simulink model "pid_simulink_with_r_and_d"  (R2015a)
settings: Solver=ode45  SolverMode=SingleTasking  StartTime=0.0  StopTime=simu.time  RelTol=1e-3
values from neighbouring files (symbols this model uses):
  plant = tf([10],[tau 1])    [mpc_period_with_abitary_reference.m]
undefined symbols (not defined in the file or in its folder): plant_ref, simu
libraries: simulink x1
settings Model: CovSFcnEnable=off  ExtModeTrigMode=oneshot  ExtModeArmWhenConnect=off  Creator=The MathWorks Inc.  LastModifiedBy=Xiaotian
settings DataIOCC: LimitDataPoints=off  SaveOutput=off  SignalLogging=off  DSMLogging=off  SaveTime=off  SignalLoggingName=sigsOut
settings OptimizationCC: BooleanDataType=off  ExpressionDepthLimit=2147483647  InitFltsAndDblsToZero=on
settings DebuggingCC: SaveWithParameterizedLinksMsg=none  UnderspecifiedInitializationDetection=Classic  MergeDetectMultiDrivingBlocksExec=none  SignalResolutionControl=TryResolveAllWithWarning  MultiTaskDSMMsg=warning  MultiTaskCondExecSysMsg=none  IntegerOverflowMsg=none  FcnCallInpInsideContextMsg=UseLocalSettings  StateNameClashWarn=warning  IntegerSaturationMsg=none
settings HardwareCC: TargetUnknown=on
settings GRTTargetCC: TargetFcnLib=ansi_tfl_tmw.mat  CombineOutputUpdateFcns=off  GRTInterface=on

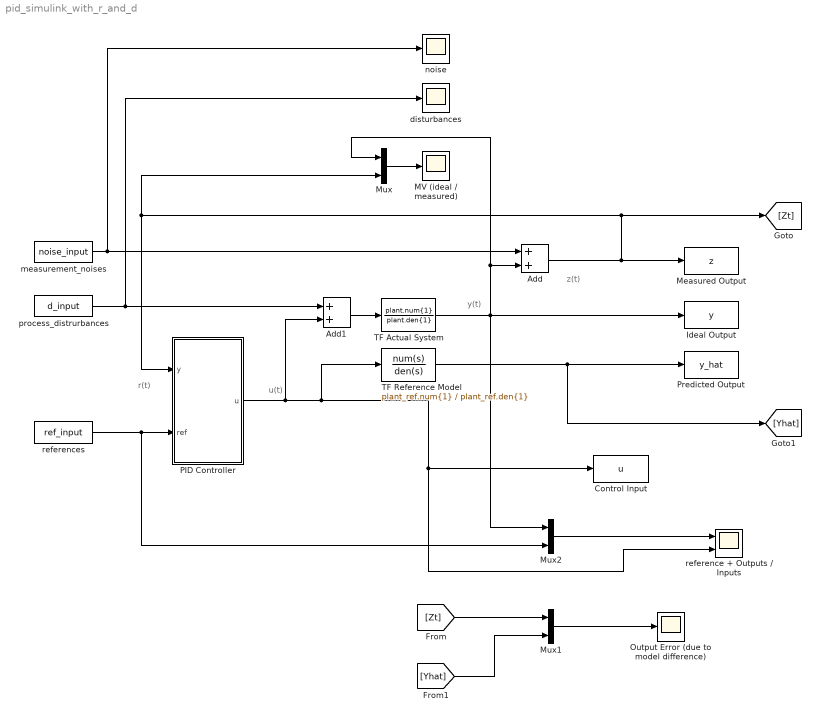
== system pid_simulink_with_r_and_d ==
  note: r(t)
  note: u(t)
  note: y(t)
  note: z(t)
  Add : Sum
  Add1 : Sum
  Control Input : ToWorkspace  VariableName=u  SampleTime=simu.samlping_time
      settings: MaxDataPoints=Inf
  Ideal Output : ToWorkspace  VariableName=y  SampleTime=simu.samlping_time
      settings: MaxDataPoints=Inf
  MV (ideal / measured) : Scope
      settings: TimeRange=10  YMin=-1.5  YMax=1.75  DataFormat=Structure
  Measured Output : ToWorkspace  VariableName=z  SampleTime=simu.samlping_time
      settings: MaxDataPoints=Inf
  Mux : Mux  Inputs=2
  Mux1 : Mux  Inputs=2
  Mux2 : Mux  Inputs=2
  Output Error (due to model difference) : Scope
      settings: TimeRange=10  YMin=-29.95  YMax=-29.6  SaveName=ScopeData2  DataFormat=Structure  SampleInput=on  SampleTime=simu.samlping_time
  PID Controller : Subsystem
  Predicted Output : ToWorkspace  VariableName=y_hat  SampleTime=simu.samlping_time
      settings: MaxDataPoints=Inf
  TF Actual System : TransferFcn  Numerator=plant.num{1}  Denominator=plant.den{1}
  TF Reference Model : TransferFcn  Numerator=plant_ref.num{1}  Denominator=plant_ref.den{1}
  disturbances : Scope
      settings: TimeRange=10  YMin=-29.95  YMax=-29.6  SaveName=ScopeData4  DataFormat=Structure  SampleInput=on  SampleTime=simu.samlping_time
  measurement_noises : FromWorkspace  VariableName=noise_input  SampleTime=0
  noise : Scope
      settings: TimeRange=10  YMin=-29.95  YMax=-29.6  SaveName=ScopeData3  DataFormat=Structure  SampleInput=on  SampleTime=simu.samlping_time
  process_distrurbances : FromWorkspace  VariableName=d_input  SampleTime=0
  reference + Outputs / Inputs : Scope  NumInputPorts=2
      settings: TimeRange=10  YMin=-2e+58~-6e+59  YMax=6.000000000000001e+58~2e+59  DataFormat=Structure  SampleInput=on  SampleTime=simu.samlping_time
  references : FromWorkspace  VariableName=ref_input  SampleTime=0
  wires:
  PID Controller/1(u) -> Add1/2, Control Input/1, reference + Outputs / Inputs/2, TF Reference Model/1
  TF Actual System/1 -> Mux2/1, Mux/1, Add/2, Ideal Output/1
  references/1 -> Mux2/2, PID Controller/2(ref)
  Add/1 -> Measured Output/1, PID Controller/1(y), Mux/2, [Zt]
  measurement_noises/1 -> noise/1, Add/1
  Add1/1 -> TF Actual System/1
  process_distrurbances/1 -> disturbances/1, Add1/1
  Mux/1 -> MV (ideal / measured)/1
  TF Reference Model/1 -> [Yhat], Predicted Output/1
  Mux1/1 -> Output Error (due to model difference)/1
  [Zt] -> Mux1/1
  [Yhat] -> Mux1/2
  Mux2/1 -> reference + Outputs / Inputs/1

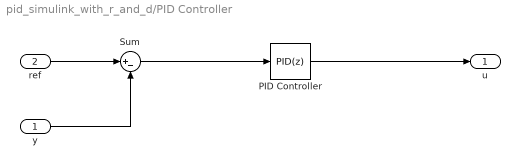
== system pid_simulink_with_r_and_d/PID Controller ==
  y : Inport
  ref : Inport  Port=2
  PID Controller : simulink/Continuous/PID Controller  Controller=PID  TimeDomain=Discrete-time  SampleTime=0.035  IntegratorMethod=Forward Euler  FilterMethod=Forward Euler  Form=Parallel  UseFilter=on  ControllerParametersSource=internal  P=10  I=1  D=0  N=10  InitialConditionSource=internal  InitialConditionForIntegrator=0  InitialConditionForFilter=0  ExternalReset=none  LimitOutput=off  UpperSaturationLimit=inf  LowerSaturationLimit=-inf  LinearizeAsGain=on  AntiWindupMode=none  Kb=1  TrackingMode=off  Kt=1  PParamMin=[]  PParamMax=[]  IParamMin=[]  IParamMax=[]  DParamMin=[]  DParamMax=[]  NParamMin=[]  NParamMax=[]  KbParamMin=[]  KbParamMax=[]  KtParamMin=[]  KtParamMax=[]  POutMin=[]  POutMax=[]  IOutMin=[]  IOutMax=[]  DOutMin=[]  DOutMax=[]  NOutMin=[]  NOutMax=[]  KbOutMin=[]  KbOutMax=[]  KtOutMin=[]  KtOutMax=[]  IntegratorOutMin=[]  IntegratorOutMax=[]  FilterOutMin=[]  FilterOutMax=[]  SumOutMin=[]  SumOutMax=[]  SumI1OutMin=[]  SumI1OutMax=[]  SumI2OutMin=[]  SumI2OutMax=[]  SumI3OutMin=[]  SumI3OutMax=[]  SumDOutMin=[]  SumDOutMax=[]  SaturationOutMin=[]  SaturationOutMax=[]  IntegratorContinuousStateAttributes=''  IntegratorStateMustResolveToSignalObject=off  IntegratorRTWStateStorageClass=Auto  FilterContinuousStateAttributes=''  FilterStateMustResolveToSignalObject=off  FilterRTWStateStorageClass=Auto  DifferentiatorICPrevScaledInput=0  DifferentiatorOutMin=[]  DifferentiatorOutMax=[]
  Sum : Sum  Inputs=|+-
  u : Outport
  wires:
  PID Controller/1 -> u/1
  ref/1 -> Sum/1
  Sum/1 -> PID Controller/1
  y/1 -> Sum/2
